simulink model "AI_Compare_2level"  (R2024b)
settings: Solver=ode1  StartTime=0.0  StopTime=4.5  FixedStep=Ts  RelTol=1e-3
PreLoadFcn:
  | Net_improve_init;L=Lac_MV;Tctrl=Ts;
PostLoadFcn:
  | Net_improve_init;L=Lac_MV;Tctrl=Ts;
InitFcn:
  | Net_improve_init;L=Lac_MV;Tctrl=Ts;
undefined symbols (not defined in the file or in its folder): C1, dend, DiscIntNeverNeededParam, f_cari, fs, Lac_MV, numd, Pref, R1, Rac_MV, Ts, Vac_peak_MV, Vdc
libraries: spsControlledVoltageSourceLib x28, powerlib_extras x25, spsGroundLib x14, spsControlledCurrentSourceLib x12, spsCurrentMeasurementLib x11, spsSeriesRLCBranchLib x7, spsThreePhaseVIMeasurementLib x6, spsIdealSwitchLib x5, spsPower3phInstantaneousLib x5, simulink x5, spsVoltageMeasurementLib x3, spsUniversalBridgeLib x1
(part 4 of 4)

== matlab function AI_Compare_2level/MATLAB Function1 ==
  data: u input; dz output
function dz = phnode_forward(u)
    % =========================================================
    % 0. 声明持久化变量 (仅在 t=0 时加载和计算一次)
    % =========================================================
    persistent W00 b00 W01 b01 W10 b10 W11 b11 W20 b20 W21 b21 W3 b3 p
    
    if isempty(W00)

        w = coder.load('2level_pHNODE_weights.mat');
        
        W00 = double(w.R_module_net_0_0_weight); b00 = double(w.R_module_net_0_0_bias(:));
        W01 = double(w.R_module_net_0_1_weight(:)); b01 = double(w.R_module_net_0_1_bias(:));
        
        W10 = double(w.R_module_net_1_0_weight); b10 = double(w.R_module_net_1_0_bias(:));
        W11 = double(w.R_module_net_1_1_weight(:)); b11 = double(w.R_module_net_1_1_bias(:));
        
        W20 = double(w.R_module_net_2_0_weight); b20 = double(w.R_module_net_2_0_bias(:));
        W21 = double(w.R_module_net_2_1_weight(:)); b21 = double(w.R_module_net_2_1_bias(:));
        
        W3  = double(w.R_module_net_3_weight);   b3  = double(w.R_module_net_3_bias(:));

        p_raw = double(w.Pinv_module_p_raw(:));
        base_scale = [1/3.3e-3; 1/3.3e-3; 1/0.015; 1/0.015; 1/0.015];
        p = log(1.0 + exp(p_raw)) .* base_scale;
    end
    
    % =========================================================
    % 1. 拆解输入向量
    % =========================================================
    z     = double(u(1:5));
    u_ext = double(u(6:10));
    u_sw  = double(u(11:16));
    
    % =========================================================
    % 2. 构造耗散矩阵 R
    % =========================================================
    h = [z; u_sw];
    
    % --- Block 0 ---
    h = W00 * h + b00;
    mu = mean(h); var_h = mean((h - mu).^2);
    h = (h - mu) ./ sqrt(var_h + 1e-5);
    h = W01 .* h + b01;
    h = h ./ (1 + exp(-h)); % SiLU
    
    % --- Block 1 ---    
    h = W10 * h + b10;
    mu = mean(h); var_h = mean((h - mu).^2);
    h = (h - mu) ./ sqrt(var_h + 1e-5);
    h = W11 .* h + b11;
    h = h ./ (1 + exp(-h));
    
    % --- Block 2 ---
    h = W20 * h + b20;
    mu = mean(h); var_h = mean((h - mu).^2);
    h = (h - mu) ./ sqrt(var_h + 1e-5);
    h = W21 .* h + b21;
    h = h ./ (1 + exp(-h));
    
    % --- Output Linear ---
    r_out = W3 * h + b3;   
    r_full = log(1 + exp(r_out)); 
    
    % =========================================================
    % 3. 计算最终输出 dz 稀疏运算
    % =========================================================
    Jz = zeros(5, 1, 'double');
    Jz(1) =  u_sw(1)*z(3) + u_sw(3)*z(4) + u_sw(5)*z(5);
    Jz(2) = -u_sw(2)*z(3) - u_sw(4)*z(4) - u_sw(6)*z(5);
    Jz(3) = -u_sw(1)*z(1) + u_sw(2)*z(2);
    Jz(4) = -u_sw(3)*z(1) + u_sw(4)*z(2);
    Jz(5) = -u_sw(5)*z(1) + u_sw(6)*z(2);
 
    rhs = Jz - r_full .* z + u_ext;
 
    dz = p .* rhs;
end
